simulink library "sm_trackV_lib_chain_contact_s46"  (R2026a)
settings: Solver=VariableStepAuto
undefined symbols (not defined in the file): Excv, L1, L10, L11, L12, L13, L14, L15, L16, L17, L18, L19, L2, L20, L21, L22, L23, L24, L25, L26, L27, L28, L29, L3, L30, L31, L32, L33, L34, L35, L36, L37, L38, L39, L4, L40, L41, L42, L43, L44, L45, L46, L5, L6, L7, L8, L9
libraries: sm_trackV_lib_chain_contact x276
Description:
  | Copyright 2024-2026 The MathWorks, Inc.
settings Model: Creator=smiller  LastModifiedBy=smiller

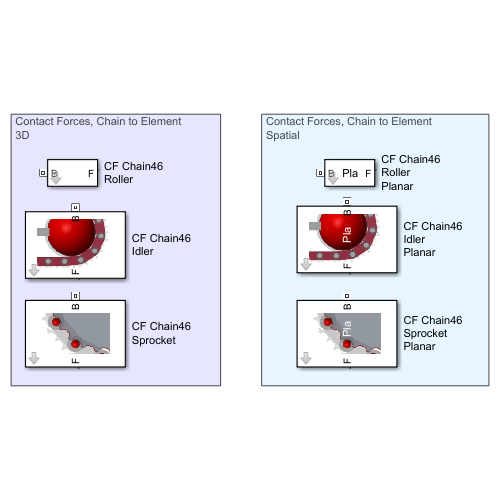
[thumbnail: Simulink's stored preview of the top-level diagram]
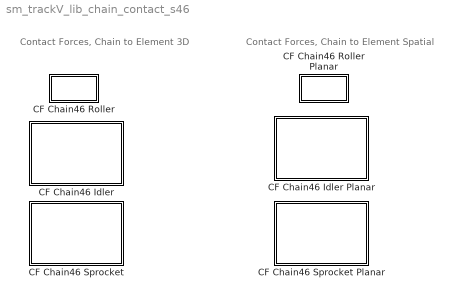
== system sm_trackV_lib_chain_contact_s46 ==
  note: Contact Forces, Chain to Element
      | 3D
  note: Contact Forces, Chain to Element
      | Spatial
  CF Chain46 Idler : Subsystem  mask(Contact Force, Full Chain to Idler){K_Idler=Excv.Contact.Idler.K, B_Idler=Excv.Contact.Idler.B, TW_Idler=Excv.Contact.Idler.TW}
      mask prompts: K_Idler "Normal Stiffness (N/m)"; B_Idler "Normal Damping (N/(m/s))"; TW_Idler "Normal Transition Width (m)"
      mask help: Models contact forces between entire chain and idler.
      mask Display: image('sm_excv_track_cf_chain_idler_IMAGE.png');
  CF Chain46 Idler Planar : Subsystem  mask(Contact Force, Full Chain to Idler){K_Idler=Excv.Contact.Idler.K, B_Idler=Excv.Contact.Idler.B, TW_Idler=Excv.Contact.Idler.TW}
      mask prompts: K_Idler "Normal Stiffness (N/m)"; B_Idler "Normal Damping (N/(m/s))"; TW_Idler "Normal Transition Width (m)"
      mask help: Models contact forces between entire chain and idler.
      mask Display:
      | image('sm_excv_track_cf_chain_idler_IMAGE.png');
      | color('white')
      | disp('   Pla');
  CF Chain46 Roller : Subsystem  mask(Contact Force, Full Chain to One Roller){K_Roller=Excv.Contact.Roller.K, B_Roller=Excv.Contact.Roller.B, TW_Roller=Excv.Contact.Roller.TW}
      mask prompts: K_Roller "Normal Stiffness (N/m)"; B_Roller "Normal Damping (N/(m/s))"; TW_Roller "Normal Transition Width (m)"
      mask help: Models contact forces between entire chain and one roller.
  CF Chain46 Roller Planar : Subsystem  mask(Contact Force, Full Chain to One Roller){K_Roller=Excv.Contact.Roller.K, B_Roller=Excv.Contact.Roller.B, TW_Roller=Excv.Contact.Roller.TW}
      mask prompts: K_Roller "Normal Stiffness (N/m)"; B_Roller "Normal Damping (N/(m/s))"; TW_Roller "Normal Transition Width (m)"
      mask help: Models contact forces between entire chain and one roller.
      mask Display: disp('Pla');
  CF Chain46 Sprocket : Subsystem  mask(Contact Force, Full Chain to Sprocket){K_Sprocket=Excv.Contact.Sprocket.K, B_Sprocket=Excv.Contact.Sprocket.B, TW_Sprocket=Excv.Contact.Sprocket.TW}
      mask prompts: K_Sprocket "Normal Stiffness (N/m)"; B_Sprocket "Normal Damping (N/(m/s))"; TW_Sprocket "Normal Transition Width (m)"
      mask help: Models contact forces between entire chain and sprocket.
      mask Display: image('sm_excv_track_cf_chain_teeth_IMAGE.png')
  CF Chain46 Sprocket Planar : Subsystem  mask(Contact Force, Full Chain to Sprocket){K_Sprocket=Excv.Contact.Sprocket.K, B_Sprocket=Excv.Contact.Sprocket.B, TW_Sprocket=Excv.Contact.Sprocket.TW}
      mask prompts: K_Sprocket "Normal Stiffness (N/m)"; B_Sprocket "Normal Damping (N/(m/s))"; TW_Sprocket "Normal Transition Width (m)"
      mask help: Models contact forces between entire chain and sprocket.
      mask Display:
      | image('sm_excv_track_cf_chain_teeth_IMAGE.png')
      | color('white')
      | disp('   Pla');

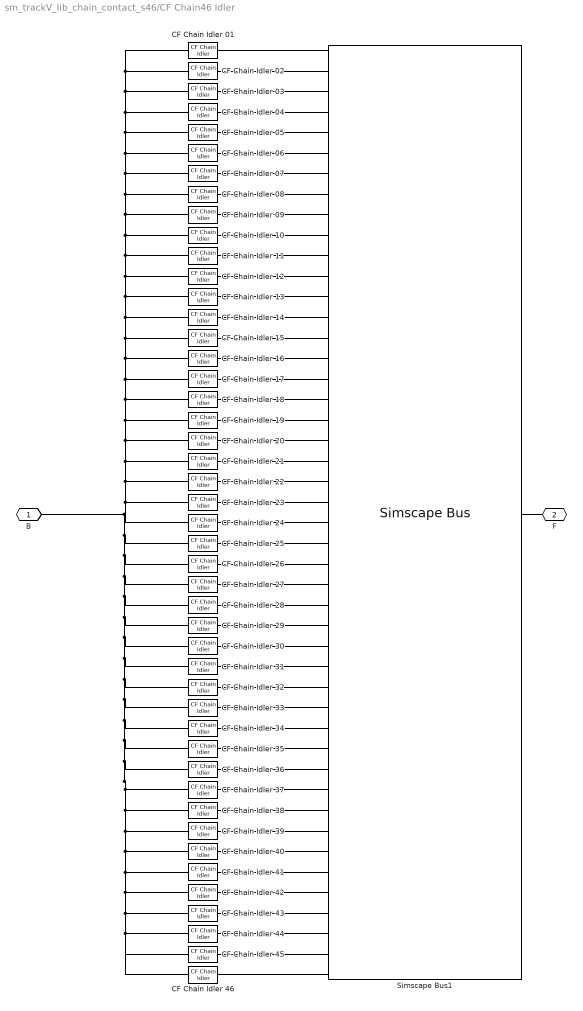
== system sm_trackV_lib_chain_contact_s46/CF Chain46 Idler ==
  CF Chain Idler 01 : sm_trackV_lib_chain_contact/CF Chain Idler  NormalStiffness=K_Idler  NormalDamping=B_Idler  NormalTransitionRegionWidth=TW_Idler
      settings: LibrarySourceBlock=sm_chain_drive_lib/CF_Idler
  CF Chain Idler 02 : sm_trackV_lib_chain_contact/CF Chain Idler  NormalStiffness=K_Idler  NormalDamping=B_Idler  NormalTransitionRegionWidth=TW_Idler
      settings: LibrarySourceBlock=sm_chain_drive_lib/CF_Idler
  CF Chain Idler 03 : sm_trackV_lib_chain_contact/CF Chain Idler  NormalStiffness=K_Idler  NormalDamping=B_Idler  NormalTransitionRegionWidth=TW_Idler
      settings: LibrarySourceBlock=sm_chain_drive_lib/CF_Idler
  CF Chain Idler 04 : sm_trackV_lib_chain_contact/CF Chain Idler  NormalStiffness=K_Idler  NormalDamping=B_Idler  NormalTransitionRegionWidth=TW_Idler
      settings: LibrarySourceBlock=sm_chain_drive_lib/CF_Idler
  CF Chain Idler 05 : sm_trackV_lib_chain_contact/CF Chain Idler  NormalStiffness=K_Idler  NormalDamping=B_Idler  NormalTransitionRegionWidth=TW_Idler
      settings: LibrarySourceBlock=sm_chain_drive_lib/CF_Idler
  CF Chain Idler 06 : sm_trackV_lib_chain_contact/CF Chain Idler  NormalStiffness=K_Idler  NormalDamping=B_Idler  NormalTransitionRegionWidth=TW_Idler
      settings: LibrarySourceBlock=sm_chain_drive_lib/CF_Idler
  CF Chain Idler 07 : sm_trackV_lib_chain_contact/CF Chain Idler  NormalStiffness=K_Idler  NormalDamping=B_Idler  NormalTransitionRegionWidth=TW_Idler
      settings: LibrarySourceBlock=sm_chain_drive_lib/CF_Idler
  CF Chain Idler 08 : sm_trackV_lib_chain_contact/CF Chain Idler  NormalStiffness=K_Idler  NormalDamping=B_Idler  NormalTransitionRegionWidth=TW_Idler
      settings: LibrarySourceBlock=sm_chain_drive_lib/CF_Idler
  CF Chain Idler 09 : sm_trackV_lib_chain_contact/CF Chain Idler  NormalStiffness=K_Idler  NormalDamping=B_Idler  NormalTransitionRegionWidth=TW_Idler
      settings: LibrarySourceBlock=sm_chain_drive_lib/CF_Idler
  CF Chain Idler {10..46} (37 alike) : sm_trackV_lib_chain_contact/CF Chain Idler  NormalStiffness=K_Idler  NormalDamping=B_Idler  NormalTransitionRegionWidth=TW_Idler
      settings: LibrarySourceBlock=sm_chain_drive_lib/CF_Idler
  Simscape Bus1 : SimscapeBus  HierarchyStrings=L1;L2;L3;L4;L5;L6;L7;L8;L9;L10;L11;L12;L13;L14;L15;L16;L17;L18;L19;L20;L21;L22;L23;L24;L25;L26;L27;L28;L29;L30;L31;L32;L33;L34;L35;L36;L37;L38;L39;L40;L41;L42;L43;L44;L45;L46  ConnectionType=Bus: CBO_Chain46
  B : PMIOPort  Side=Left
  F : PMIOPort  Port=2  Side=Right
  connections:
  Simscape Bus1/RConn1 -- F/RConn1
  Simscape Bus1/LConn28 -- CF Chain Idler 28/RConn1
  Simscape Bus1/LConn27 -- CF Chain Idler 27/RConn1
  Simscape Bus1/LConn26 -- CF Chain Idler 26/RConn1
  Simscape Bus1/LConn25 -- CF Chain Idler 25/RConn1
  Simscape Bus1/LConn24 -- CF Chain Idler 24/RConn1
  Simscape Bus1/LConn23 -- CF Chain Idler 23/RConn1
  Simscape Bus1/LConn22 -- CF Chain Idler 22/RConn1
  Simscape Bus1/LConn21 -- CF Chain Idler 21/RConn1
  Simscape Bus1/LConn20 -- CF Chain Idler 20/RConn1
  Simscape Bus1/LConn19 -- CF Chain Idler 19/RConn1
  Simscape Bus1/LConn18 -- CF Chain Idler 18/RConn1
  Simscape Bus1/LConn17 -- CF Chain Idler 17/RConn1
  Simscape Bus1/LConn16 -- CF Chain Idler 16/RConn1
  Simscape Bus1/LConn15 -- CF Chain Idler 15/RConn1
  Simscape Bus1/LConn14 -- CF Chain Idler 14/RConn1
  Simscape Bus1/LConn13 -- CF Chain Idler 13/RConn1
  Simscape Bus1/LConn12 -- CF Chain Idler 12/RConn1
  Simscape Bus1/LConn11 -- CF Chain Idler 11/RConn1
  Simscape Bus1/LConn10 -- CF Chain Idler 10/RConn1
  Simscape Bus1/LConn9 -- CF Chain Idler 09/RConn1
  Simscape Bus1/LConn8 -- CF Chain Idler 08/RConn1
  Simscape Bus1/LConn7 -- CF Chain Idler 07/RConn1
  Simscape Bus1/LConn6 -- CF Chain Idler 06/RConn1
  Simscape Bus1/LConn5 -- CF Chain Idler 05/RConn1
  Simscape Bus1/LConn4 -- CF Chain Idler 04/RConn1
  Simscape Bus1/LConn3 -- CF Chain Idler 03/RConn1
  Simscape Bus1/LConn2 -- CF Chain Idler 02/RConn1
  Simscape Bus1/LConn1 -- CF Chain Idler 01/RConn1
  CF Chain Idler 02/LConn1 -- CF Chain Idler 01/LConn1 -- CF Chain Idler 03/LConn1 -- CF Chain Idler 04/LConn1 -- CF Chain Idler 05/LConn1 -- CF Chain Idler 06/LConn1 -- CF Chain Idler 07/LConn1 -- CF Chain Idler 08/LConn1 -- CF Chain Idler 09/LConn1 -- CF Chain Idler 10/LConn1 -- CF Chain Idler 11/LConn1 -- CF Chain Idler 12/LConn1 -- CF Chain Idler 13/LConn1 -- CF Chain Idler 14/LConn1 -- CF Chain Idler 15/LConn1 -- CF Chain Idler 16/LConn1 -- CF Chain Idler 17/LConn1 -- CF Chain Idler 18/LConn1 -- CF Chain Idler 19/LConn1 -- CF Chain Idler 20/LConn1 -- CF Chain Idler 21/LConn1 -- CF Chain Idler 22/LConn1 -- CF Chain Idler 23/LConn1 -- B/RConn1 -- CF Chain Idler 24/LConn1 -- CF Chain Idler 25/LConn1 -- CF Chain Idler 26/LConn1 -- CF Chain Idler 27/LConn1 -- CF Chain Idler 28/LConn1 -- CF Chain Idler 29/LConn1 -- CF Chain Idler 30/LConn1 -- CF Chain Idler 31/LConn1 -- CF Chain Idler 32/LConn1 -- CF Chain Idler 33/LConn1 -- CF Chain Idler 34/LConn1 -- CF Chain Idler 35/LConn1 -- CF Chain Idler 36/LConn1 -- CF Chain Idler 37/LConn1 -- CF Chain Idler 38/LConn1 -- CF Chain Idler 39/LConn1 -- CF Chain Idler 40/LConn1 -- CF Chain Idler 41/LConn1 -- CF Chain Idler 42/LConn1 -- CF Chain Idler 43/LConn1 -- CF Chain Idler 44/LConn1 -- CF Chain Idler 46/LConn1 -- CF Chain Idler 45/LConn1
  Simscape Bus1/LConn46 -- CF Chain Idler 46/RConn1
  Simscape Bus1/LConn45 -- CF Chain Idler 45/RConn1
  Simscape Bus1/LConn44 -- CF Chain Idler 44/RConn1
  Simscape Bus1/LConn43 -- CF Chain Idler 43/RConn1
  Simscape Bus1/LConn42 -- CF Chain Idler 42/RConn1
  Simscape Bus1/LConn41 -- CF Chain Idler 41/RConn1
  Simscape Bus1/LConn40 -- CF Chain Idler 40/RConn1
  Simscape Bus1/LConn39 -- CF Chain Idler 39/RConn1
  Simscape Bus1/LConn38 -- CF Chain Idler 38/RConn1
  Simscape Bus1/LConn37 -- CF Chain Idler 37/RConn1
  Simscape Bus1/LConn36 -- CF Chain Idler 36/RConn1
  Simscape Bus1/LConn35 -- CF Chain Idler 35/RConn1
  Simscape Bus1/LConn34 -- CF Chain Idler 34/RConn1
  Simscape Bus1/LConn33 -- CF Chain Idler 33/RConn1
  Simscape Bus1/LConn32 -- CF Chain Idler 32/RConn1
  Simscape Bus1/LConn31 -- CF Chain Idler 31/RConn1
  Simscape Bus1/LConn30 -- CF Chain Idler 30/RConn1
  Simscape Bus1/LConn29 -- CF Chain Idler 29/RConn1

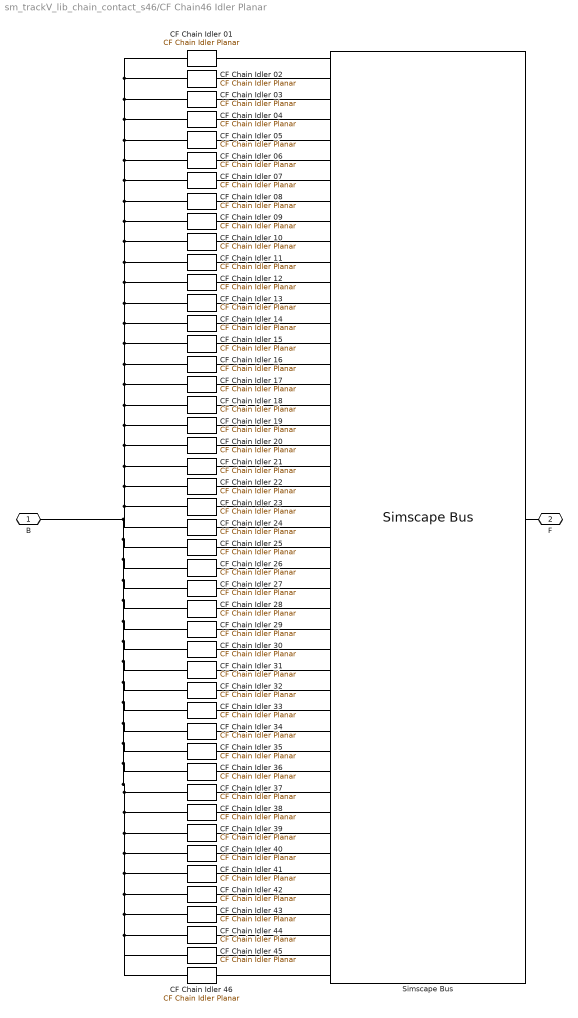
== system sm_trackV_lib_chain_contact_s46/CF Chain46 Idler Planar ==
  CF Chain Idler 01 : sm_trackV_lib_chain_contact/CF Chain Idler Planar  NormalStiffness=K_Idler  NormalDamping=B_Idler  NormalTransitionRegionWidth=TW_Idler
  CF Chain Idler 02 : sm_trackV_lib_chain_contact/CF Chain Idler Planar  NormalStiffness=K_Idler  NormalDamping=B_Idler  NormalTransitionRegionWidth=TW_Idler
  CF Chain Idler 03 : sm_trackV_lib_chain_contact/CF Chain Idler Planar  NormalStiffness=K_Idler  NormalDamping=B_Idler  NormalTransitionRegionWidth=TW_Idler
  CF Chain Idler 04 : sm_trackV_lib_chain_contact/CF Chain Idler Planar  NormalStiffness=K_Idler  NormalDamping=B_Idler  NormalTransitionRegionWidth=TW_Idler
  CF Chain Idler 05 : sm_trackV_lib_chain_contact/CF Chain Idler Planar  NormalStiffness=K_Idler  NormalDamping=B_Idler  NormalTransitionRegionWidth=TW_Idler
  CF Chain Idler 06 : sm_trackV_lib_chain_contact/CF Chain Idler Planar  NormalStiffness=K_Idler  NormalDamping=B_Idler  NormalTransitionRegionWidth=TW_Idler
  CF Chain Idler 07 : sm_trackV_lib_chain_contact/CF Chain Idler Planar  NormalStiffness=K_Idler  NormalDamping=B_Idler  NormalTransitionRegionWidth=TW_Idler
  CF Chain Idler 08 : sm_trackV_lib_chain_contact/CF Chain Idler Planar  NormalStiffness=K_Idler  NormalDamping=B_Idler  NormalTransitionRegionWidth=TW_Idler
  CF Chain Idler 09 : sm_trackV_lib_chain_contact/CF Chain Idler Planar  NormalStiffness=K_Idler  NormalDamping=B_Idler  NormalTransitionRegionWidth=TW_Idler
  CF Chain Idler {10..46} (37 alike) : sm_trackV_lib_chain_contact/CF Chain Idler Planar  NormalStiffness=K_Idler  NormalDamping=B_Idler  NormalTransitionRegionWidth=TW_Idler
  Simscape Bus : SimscapeBus  HierarchyStrings=L1;L2;L3;L4;L5;L6;L7;L8;L9;L10;L11;L12;L13;L14;L15;L16;L17;L18;L19;L20;L21;L22;L23;L24;L25;L26;L27;L28;L29;L30;L31;L32;L33;L34;L35;L36;L37;L38;L39;L40;L41;L42;L43;L44;L45;L46  ConnectionType=Bus: CBO_Chain46
  B : PMIOPort  Side=Left
  F : PMIOPort  Port=2  Side=Right
  connections:
  Simscape Bus/RConn1 -- F/RConn1
  CF Chain Idler 28/RConn1 -- Simscape Bus/LConn28
  CF Chain Idler 27/RConn1 -- Simscape Bus/LConn27
  CF Chain Idler 26/RConn1 -- Simscape Bus/LConn26
  CF Chain Idler 25/RConn1 -- Simscape Bus/LConn25
  CF Chain Idler 24/RConn1 -- Simscape Bus/LConn24
  CF Chain Idler 23/RConn1 -- Simscape Bus/LConn23
  CF Chain Idler 22/RConn1 -- Simscape Bus/LConn22
  CF Chain Idler 21/RConn1 -- Simscape Bus/LConn21
  CF Chain Idler 20/RConn1 -- Simscape Bus/LConn20
  CF Chain Idler 19/RConn1 -- Simscape Bus/LConn19
  CF Chain Idler 18/RConn1 -- Simscape Bus/LConn18
  CF Chain Idler 17/RConn1 -- Simscape Bus/LConn17
  CF Chain Idler 16/RConn1 -- Simscape Bus/LConn16
  CF Chain Idler 15/RConn1 -- Simscape Bus/LConn15
  CF Chain Idler 14/RConn1 -- Simscape Bus/LConn14
  CF Chain Idler 13/RConn1 -- Simscape Bus/LConn13
  CF Chain Idler 12/RConn1 -- Simscape Bus/LConn12
  CF Chain Idler 11/RConn1 -- Simscape Bus/LConn11
  CF Chain Idler 10/RConn1 -- Simscape Bus/LConn10
  CF Chain Idler 09/RConn1 -- Simscape Bus/LConn9
  CF Chain Idler 08/RConn1 -- Simscape Bus/LConn8
  CF Chain Idler 07/RConn1 -- Simscape Bus/LConn7
  CF Chain Idler 06/RConn1 -- Simscape Bus/LConn6
  CF Chain Idler 05/RConn1 -- Simscape Bus/LConn5
  CF Chain Idler 04/RConn1 -- Simscape Bus/LConn4
  CF Chain Idler 03/RConn1 -- Simscape Bus/LConn3
  CF Chain Idler 02/RConn1 -- Simscape Bus/LConn2
  CF Chain Idler 01/RConn1 -- Simscape Bus/LConn1
  CF Chain Idler 02/LConn1 -- CF Chain Idler 01/LConn1 -- CF Chain Idler 03/LConn1 -- CF Chain Idler 04/LConn1 -- CF Chain Idler 05/LConn1 -- CF Chain Idler 06/LConn1 -- CF Chain Idler 07/LConn1 -- CF Chain Idler 08/LConn1 -- CF Chain Idler 09/LConn1 -- CF Chain Idler 10/LConn1 -- CF Chain Idler 11/LConn1 -- CF Chain Idler 12/LConn1 -- CF Chain Idler 13/LConn1 -- CF Chain Idler 14/LConn1 -- CF Chain Idler 15/LConn1 -- CF Chain Idler 16/LConn1 -- CF Chain Idler 17/LConn1 -- CF Chain Idler 18/LConn1 -- CF Chain Idler 19/LConn1 -- CF Chain Idler 20/LConn1 -- CF Chain Idler 21/LConn1 -- CF Chain Idler 22/LConn1 -- CF Chain Idler 23/LConn1 -- B/RConn1 -- CF Chain Idler 24/LConn1 -- CF Chain Idler 25/LConn1 -- CF Chain Idler 26/LConn1 -- CF Chain Idler 27/LConn1 -- CF Chain Idler 28/LConn1 -- CF Chain Idler 29/LConn1 -- CF Chain Idler 30/LConn1 -- CF Chain Idler 31/LConn1 -- CF Chain Idler 32/LConn1 -- CF Chain Idler 33/LConn1 -- CF Chain Idler 34/LConn1 -- CF Chain Idler 35/LConn1 -- CF Chain Idler 36/LConn1 -- CF Chain Idler 37/LConn1 -- CF Chain Idler 38/LConn1 -- CF Chain Idler 39/LConn1 -- CF Chain Idler 40/LConn1 -- CF Chain Idler 41/LConn1 -- CF Chain Idler 42/LConn1 -- CF Chain Idler 43/LConn1 -- CF Chain Idler 44/LConn1 -- CF Chain Idler 46/LConn1 -- CF Chain Idler 45/LConn1
  CF Chain Idler 46/RConn1 -- Simscape Bus/LConn46
  CF Chain Idler 45/RConn1 -- Simscape Bus/LConn45
  CF Chain Idler 44/RConn1 -- Simscape Bus/LConn44
  CF Chain Idler 43/RConn1 -- Simscape Bus/LConn43
  CF Chain Idler 42/RConn1 -- Simscape Bus/LConn42
  CF Chain Idler 41/RConn1 -- Simscape Bus/LConn41
  CF Chain Idler 40/RConn1 -- Simscape Bus/LConn40
  CF Chain Idler 39/RConn1 -- Simscape Bus/LConn39
  CF Chain Idler 38/RConn1 -- Simscape Bus/LConn38
  CF Chain Idler 37/RConn1 -- Simscape Bus/LConn37
  CF Chain Idler 36/RConn1 -- Simscape Bus/LConn36
  CF Chain Idler 35/RConn1 -- Simscape Bus/LConn35
  CF Chain Idler 34/RConn1 -- Simscape Bus/LConn34
  CF Chain Idler 33/RConn1 -- Simscape Bus/LConn33
  CF Chain Idler 32/RConn1 -- Simscape Bus/LConn32
  CF Chain Idler 31/RConn1 -- Simscape Bus/LConn31
  CF Chain Idler 30/RConn1 -- Simscape Bus/LConn30
  CF Chain Idler 29/RConn1 -- Simscape Bus/LConn29

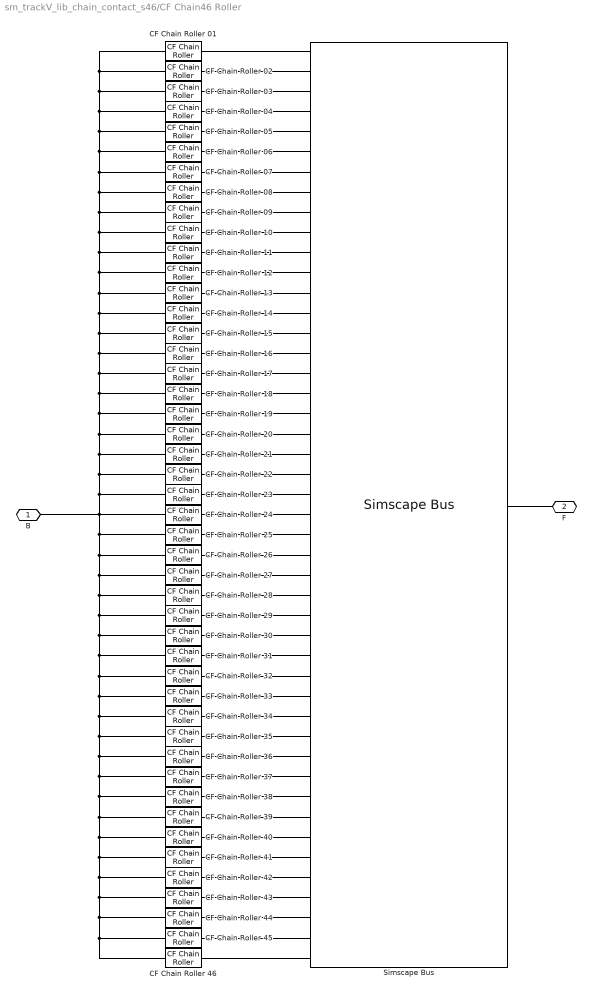
== system sm_trackV_lib_chain_contact_s46/CF Chain46 Roller ==
  CF Chain Roller 01 : sm_trackV_lib_chain_contact/CF Chain Roller  NormalStiffness=K_Roller  NormalDamping=B_Roller  NormalTransitionRegionWidth=TW_Roller
      settings: LibrarySourceBlock=sm_chain_drive_lib/CF_Pulley
  CF Chain Roller 02 : sm_trackV_lib_chain_contact/CF Chain Roller  NormalStiffness=K_Roller  NormalDamping=B_Roller  NormalTransitionRegionWidth=TW_Roller
      settings: LibrarySourceBlock=sm_chain_drive_lib/CF_Pulley
  CF Chain Roller 03 : sm_trackV_lib_chain_contact/CF Chain Roller  NormalStiffness=K_Roller  NormalDamping=B_Roller  NormalTransitionRegionWidth=TW_Roller
      settings: LibrarySourceBlock=sm_chain_drive_lib/CF_Pulley
  CF Chain Roller 04 : sm_trackV_lib_chain_contact/CF Chain Roller  NormalStiffness=K_Roller  NormalDamping=B_Roller  NormalTransitionRegionWidth=TW_Roller
      settings: LibrarySourceBlock=sm_chain_drive_lib/CF_Pulley
  CF Chain Roller 05 : sm_trackV_lib_chain_contact/CF Chain Roller  NormalStiffness=K_Roller  NormalDamping=B_Roller  NormalTransitionRegionWidth=TW_Roller
      settings: LibrarySourceBlock=sm_chain_drive_lib/CF_Pulley
  CF Chain Roller 06 : sm_trackV_lib_chain_contact/CF Chain Roller  NormalStiffness=K_Roller  NormalDamping=B_Roller  NormalTransitionRegionWidth=TW_Roller
      settings: LibrarySourceBlock=sm_chain_drive_lib/CF_Pulley
  CF Chain Roller 07 : sm_trackV_lib_chain_contact/CF Chain Roller  NormalStiffness=K_Roller  NormalDamping=B_Roller  NormalTransitionRegionWidth=TW_Roller
      settings: LibrarySourceBlock=sm_chain_drive_lib/CF_Pulley
  CF Chain Roller 08 : sm_trackV_lib_chain_contact/CF Chain Roller  NormalStiffness=K_Roller  NormalDamping=B_Roller  NormalTransitionRegionWidth=TW_Roller
      settings: LibrarySourceBlock=sm_chain_drive_lib/CF_Pulley
  CF Chain Roller 09 : sm_trackV_lib_chain_contact/CF Chain Roller  NormalStiffness=K_Roller  NormalDamping=B_Roller  NormalTransitionRegionWidth=TW_Roller
      settings: LibrarySourceBlock=sm_chain_drive_lib/CF_Pulley
  CF Chain Roller {10..46} (37 alike) : sm_trackV_lib_chain_contact/CF Chain Roller  NormalStiffness=K_Roller  NormalDamping=B_Roller  NormalTransitionRegionWidth=TW_Roller
      settings: LibrarySourceBlock=sm_chain_drive_lib/CF_Pulley
  Simscape Bus : SimscapeBus  HierarchyStrings=L1;L2;L3;L4;L5;L6;L7;L8;L9;L10;L11;L12;L13;L14;L15;L16;L17;L18;L19;L20;L21;L22;L23;L24;L25;L26;L27;L28;L29;L30;L31;L32;L33;L34;L35;L36;L37;L38;L39;L40;L41;L42;L43;L44;L45;L46  ConnectionType=Bus: CBO_Chain46
  B : PMIOPort  Side=Left
  F : PMIOPort  Port=2  Side=Right
  connections:
  CF Chain Roller 28/RConn1 -- Simscape Bus/LConn28
  CF Chain Roller 27/RConn1 -- Simscape Bus/LConn27
  CF Chain Roller 26/RConn1 -- Simscape Bus/LConn26
  CF Chain Roller 25/RConn1 -- Simscape Bus/LConn25
  CF Chain Roller 24/RConn1 -- Simscape Bus/LConn24
  CF Chain Roller 23/RConn1 -- Simscape Bus/LConn23
  CF Chain Roller 22/RConn1 -- Simscape Bus/LConn22
  CF Chain Roller 21/RConn1 -- Simscape Bus/LConn21
  CF Chain Roller 20/RConn1 -- Simscape Bus/LConn20
  CF Chain Roller 19/RConn1 -- Simscape Bus/LConn19
  CF Chain Roller 18/RConn1 -- Simscape Bus/LConn18
  CF Chain Roller 17/RConn1 -- Simscape Bus/LConn17
  CF Chain Roller 16/RConn1 -- Simscape Bus/LConn16
  CF Chain Roller 15/RConn1 -- Simscape Bus/LConn15
  CF Chain Roller 14/RConn1 -- Simscape Bus/LConn14
  CF Chain Roller 13/RConn1 -- Simscape Bus/LConn13
  CF Chain Roller 12/RConn1 -- Simscape Bus/LConn12
  CF Chain Roller 11/RConn1 -- Simscape Bus/LConn11
  CF Chain Roller 10/RConn1 -- Simscape Bus/LConn10
  CF Chain Roller 09/RConn1 -- Simscape Bus/LConn9
  CF Chain Roller 08/RConn1 -- Simscape Bus/LConn8
  CF Chain Roller 07/RConn1 -- Simscape Bus/LConn7
  CF Chain Roller 06/RConn1 -- Simscape Bus/LConn6
  CF Chain Roller 05/RConn1 -- Simscape Bus/LConn5
  CF Chain Roller 04/RConn1 -- Simscape Bus/LConn4
  CF Chain Roller 03/RConn1 -- Simscape Bus/LConn3
  CF Chain Roller 02/RConn1 -- Simscape Bus/LConn2
  Simscape Bus/LConn1 -- CF Chain Roller 01/RConn1
  Simscape Bus/RConn1 -- F/RConn1
  CF Chain Roller 29/RConn1 -- Simscape Bus/LConn29
  CF Chain Roller 30/RConn1 -- Simscape Bus/LConn30
  CF Chain Roller 31/RConn1 -- Simscape Bus/LConn31
  CF Chain Roller 32/RConn1 -- Simscape Bus/LConn32
  CF Chain Roller 33/RConn1 -- Simscape Bus/LConn33
  CF Chain Roller 34/RConn1 -- Simscape Bus/LConn34
  CF Chain Roller 35/RConn1 -- Simscape Bus/LConn35
  CF Chain Roller 36/RConn1 -- Simscape Bus/LConn36
  CF Chain Roller 37/RConn1 -- Simscape Bus/LConn37
  CF Chain Roller 38/RConn1 -- Simscape Bus/LConn38
  CF Chain Roller 39/RConn1 -- Simscape Bus/LConn39
  CF Chain Roller 40/RConn1 -- Simscape Bus/LConn40
  CF Chain Roller 41/RConn1 -- Simscape Bus/LConn41
  CF Chain Roller 42/RConn1 -- Simscape Bus/LConn42
  CF Chain Roller 43/RConn1 -- Simscape Bus/LConn43
  CF Chain Roller 44/RConn1 -- Simscape Bus/LConn44
  CF Chain Roller 45/RConn1 -- Simscape Bus/LConn45
  CF Chain Roller 46/RConn1 -- Simscape Bus/LConn46
  B/RConn1 -- CF Chain Roller 01/LConn1 -- CF Chain Roller 02/LConn1 -- CF Chain Roller 03/LConn1 -- CF Chain Roller 04/LConn1 -- CF Chain Roller 05/LConn1 -- CF Chain Roller 06/LConn1 -- CF Chain Roller 07/LConn1 -- CF Chain Roller 08/LConn1 -- CF Chain Roller 09/LConn1 -- CF Chain Roller 10/LConn1 -- CF Chain Roller 11/LConn1 -- CF Chain Roller 12/LConn1 -- CF Chain Roller 13/LConn1 -- CF Chain Roller 14/LConn1 -- CF Chain Roller 15/LConn1 -- CF Chain Roller 16/LConn1 -- CF Chain Roller 17/LConn1 -- CF Chain Roller 18/LConn1 -- CF Chain Roller 19/LConn1 -- CF Chain Roller 20/LConn1 -- CF Chain Roller 21/LConn1 -- CF Chain Roller 22/LConn1 -- CF Chain Roller 23/LConn1 -- CF Chain Roller 24/LConn1 -- CF Chain Roller 25/LConn1 -- CF Chain Roller 26/LConn1 -- CF Chain Roller 27/LConn1 -- CF Chain Roller 28/LConn1 -- CF Chain Roller 29/LConn1 -- CF Chain Roller 30/LConn1 -- CF Chain Roller 31/LConn1 -- CF Chain Roller 32/LConn1 -- CF Chain Roller 33/LConn1 -- CF Chain Roller 34/LConn1 -- CF Chain Roller 35/LConn1 -- CF Chain Roller 36/LConn1 -- CF Chain Roller 37/LConn1 -- CF Chain Roller 38/LConn1 -- CF Chain Roller 39/LConn1 -- CF Chain Roller 40/LConn1 -- CF Chain Roller 41/LConn1 -- CF Chain Roller 42/LConn1 -- CF Chain Roller 43/LConn1 -- CF Chain Roller 44/LConn1 -- CF Chain Roller 46/LConn1 -- CF Chain Roller 45/LConn1

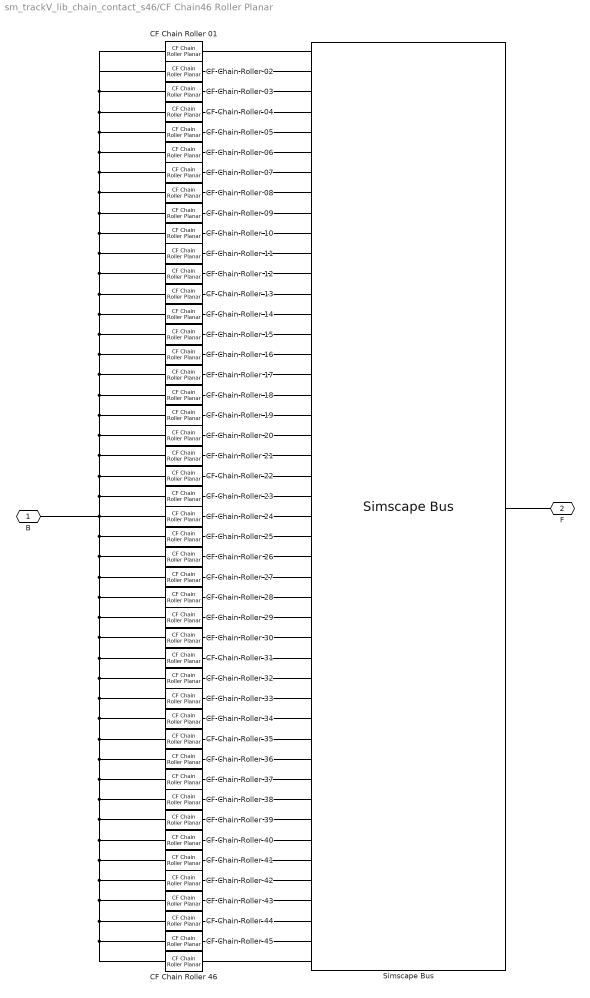
== system sm_trackV_lib_chain_contact_s46/CF Chain46 Roller Planar ==
  CF Chain Roller 01 : sm_trackV_lib_chain_contact/CF Chain Roller Planar  NormalStiffness=K_Roller  NormalDamping=B_Roller  NormalTransitionRegionWidth=TW_Roller
  CF Chain Roller 02 : sm_trackV_lib_chain_contact/CF Chain Roller Planar  NormalStiffness=K_Roller  NormalDamping=B_Roller  NormalTransitionRegionWidth=TW_Roller
  CF Chain Roller 03 : sm_trackV_lib_chain_contact/CF Chain Roller Planar  NormalStiffness=K_Roller  NormalDamping=B_Roller  NormalTransitionRegionWidth=TW_Roller
  CF Chain Roller 04 : sm_trackV_lib_chain_contact/CF Chain Roller Planar  NormalStiffness=K_Roller  NormalDamping=B_Roller  NormalTransitionRegionWidth=TW_Roller
  CF Chain Roller 05 : sm_trackV_lib_chain_contact/CF Chain Roller Planar  NormalStiffness=K_Roller  NormalDamping=B_Roller  NormalTransitionRegionWidth=TW_Roller
  CF Chain Roller 06 : sm_trackV_lib_chain_contact/CF Chain Roller Planar  NormalStiffness=K_Roller  NormalDamping=B_Roller  NormalTransitionRegionWidth=TW_Roller
  CF Chain Roller 07 : sm_trackV_lib_chain_contact/CF Chain Roller Planar  NormalStiffness=K_Roller  NormalDamping=B_Roller  NormalTransitionRegionWidth=TW_Roller
  CF Chain Roller 08 : sm_trackV_lib_chain_contact/CF Chain Roller Planar  NormalStiffness=K_Roller  NormalDamping=B_Roller  NormalTransitionRegionWidth=TW_Roller
  CF Chain Roller 09 : sm_trackV_lib_chain_contact/CF Chain Roller Planar  NormalStiffness=K_Roller  NormalDamping=B_Roller  NormalTransitionRegionWidth=TW_Roller
  CF Chain Roller {10..46} (37 alike) : sm_trackV_lib_chain_contact/CF Chain Roller Planar  NormalStiffness=K_Roller  NormalDamping=B_Roller  NormalTransitionRegionWidth=TW_Roller
  Simscape Bus : SimscapeBus  HierarchyStrings=L1;L2;L3;L4;L5;L6;L7;L8;L9;L10;L11;L12;L13;L14;L15;L16;L17;L18;L19;L20;L21;L22;L23;L24;L25;L26;L27;L28;L29;L30;L31;L32;L33;L34;L35;L36;L37;L38;L39;L40;L41;L42;L43;L44;L45;L46  ConnectionType=Bus: CBO_Chain46
  B : PMIOPort  Side=Left
  F : PMIOPort  Port=2  Side=Right
  connections:
  CF Chain Roller 45/LConn1 -- CF Chain Roller 46/LConn1 -- CF Chain Roller 44/LConn1 -- CF Chain Roller 43/LConn1 -- CF Chain Roller 42/LConn1 -- CF Chain Roller 41/LConn1 -- CF Chain Roller 40/LConn1 -- CF Chain Roller 39/LConn1 -- CF Chain Roller 38/LConn1 -- CF Chain Roller 37/LConn1 -- CF Chain Roller 36/LConn1 -- CF Chain Roller 35/LConn1 -- CF Chain Roller 34/LConn1 -- CF Chain Roller 33/LConn1 -- CF Chain Roller 32/LConn1 -- CF Chain Roller 31/LConn1 -- CF Chain Roller 30/LConn1 -- CF Chain Roller 29/LConn1 -- CF Chain Roller 28/LConn1 -- CF Chain Roller 27/LConn1 -- CF Chain Roller 26/LConn1 -- CF Chain Roller 25/LConn1 -- CF Chain Roller 24/LConn1 -- CF Chain Roller 23/LConn1 -- CF Chain Roller 22/LConn1 -- CF Chain Roller 21/LConn1 -- CF Chain Roller 20/LConn1 -- CF Chain Roller 19/LConn1 -- CF Chain Roller 18/LConn1 -- CF Chain Roller 17/LConn1 -- CF Chain Roller 16/LConn1 -- CF Chain Roller 15/LConn1 -- CF Chain Roller 14/LConn1 -- CF Chain Roller 13/LConn1 -- CF Chain Roller 12/LConn1 -- CF Chain Roller 11/LConn1 -- CF Chain Roller 10/LConn1 -- CF Chain Roller 09/LConn1 -- CF Chain Roller 08/LConn1 -- CF Chain Roller 07/LConn1 -- CF Chain Roller 06/LConn1 -- CF Chain Roller 05/LConn1 -- CF Chain Roller 04/LConn1 -- CF Chain Roller 03/LConn1 -- CF Chain Roller 02/LConn1 -- CF Chain Roller 01/LConn1 -- B/RConn1
  CF Chain Roller 46/RConn1 -- Simscape Bus/LConn46
  CF Chain Roller 45/RConn1 -- Simscape Bus/LConn45
  CF Chain Roller 44/RConn1 -- Simscape Bus/LConn44
  CF Chain Roller 43/RConn1 -- Simscape Bus/LConn43
  CF Chain Roller 42/RConn1 -- Simscape Bus/LConn42
  CF Chain Roller 41/RConn1 -- Simscape Bus/LConn41
  CF Chain Roller 40/RConn1 -- Simscape Bus/LConn40
  CF Chain Roller 39/RConn1 -- Simscape Bus/LConn39
  CF Chain Roller 38/RConn1 -- Simscape Bus/LConn38
  CF Chain Roller 37/RConn1 -- Simscape Bus/LConn37
  CF Chain Roller 36/RConn1 -- Simscape Bus/LConn36
  CF Chain Roller 35/RConn1 -- Simscape Bus/LConn35
  CF Chain Roller 34/RConn1 -- Simscape Bus/LConn34
  CF Chain Roller 33/RConn1 -- Simscape Bus/LConn33
  CF Chain Roller 32/RConn1 -- Simscape Bus/LConn32
  CF Chain Roller 31/RConn1 -- Simscape Bus/LConn31
  CF Chain Roller 30/RConn1 -- Simscape Bus/LConn30
  CF Chain Roller 29/RConn1 -- Simscape Bus/LConn29
  Simscape Bus/RConn1 -- F/RConn1
  Simscape Bus/LConn1 -- CF Chain Roller 01/RConn1
  CF Chain Roller 02/RConn1 -- Simscape Bus/LConn2
  CF Chain Roller 03/RConn1 -- Simscape Bus/LConn3
  CF Chain Roller 04/RConn1 -- Simscape Bus/LConn4
  CF Chain Roller 05/RConn1 -- Simscape Bus/LConn5
  CF Chain Roller 06/RConn1 -- Simscape Bus/LConn6
  CF Chain Roller 07/RConn1 -- Simscape Bus/LConn7
  CF Chain Roller 08/RConn1 -- Simscape Bus/LConn8
  CF Chain Roller 09/RConn1 -- Simscape Bus/LConn9
  CF Chain Roller 10/RConn1 -- Simscape Bus/LConn10
  CF Chain Roller 11/RConn1 -- Simscape Bus/LConn11
  CF Chain Roller 12/RConn1 -- Simscape Bus/LConn12
  CF Chain Roller 13/RConn1 -- Simscape Bus/LConn13
  CF Chain Roller 14/RConn1 -- Simscape Bus/LConn14
  CF Chain Roller 15/RConn1 -- Simscape Bus/LConn15
  CF Chain Roller 16/RConn1 -- Simscape Bus/LConn16
  CF Chain Roller 17/RConn1 -- Simscape Bus/LConn17
  CF Chain Roller 18/RConn1 -- Simscape Bus/LConn18
  CF Chain Roller 19/RConn1 -- Simscape Bus/LConn19
  CF Chain Roller 20/RConn1 -- Simscape Bus/LConn20
  CF Chain Roller 21/RConn1 -- Simscape Bus/LConn21
  CF Chain Roller 22/RConn1 -- Simscape Bus/LConn22
  CF Chain Roller 23/RConn1 -- Simscape Bus/LConn23
  CF Chain Roller 24/RConn1 -- Simscape Bus/LConn24
  CF Chain Roller 25/RConn1 -- Simscape Bus/LConn25
  CF Chain Roller 26/RConn1 -- Simscape Bus/LConn26
  CF Chain Roller 27/RConn1 -- Simscape Bus/LConn27
  CF Chain Roller 28/RConn1 -- Simscape Bus/LConn28

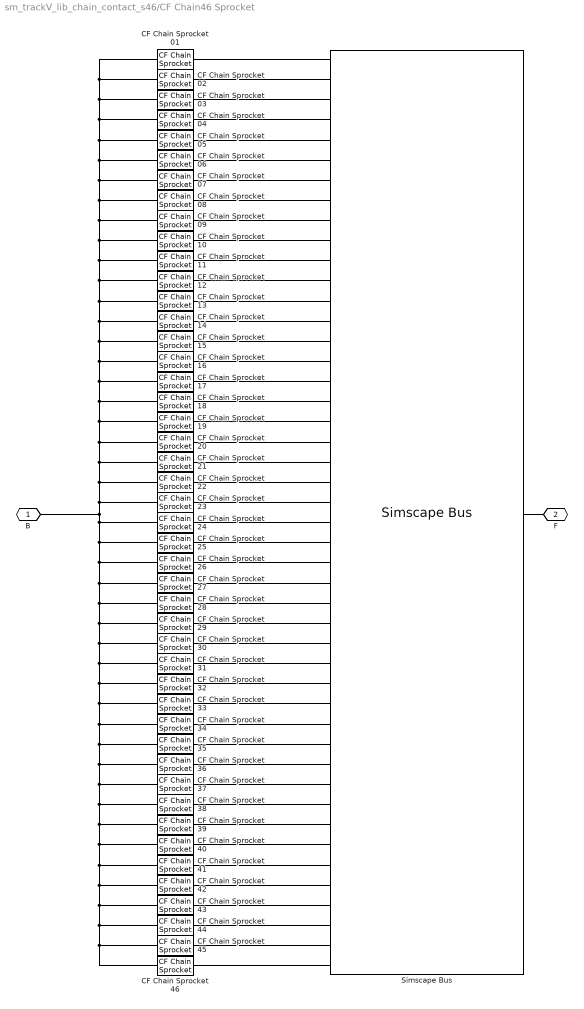
== system sm_trackV_lib_chain_contact_s46/CF Chain46 Sprocket ==
  CF Chain Sprocket 01 : sm_trackV_lib_chain_contact/CF Chain Sprocket  NormalStiffness=K_Sprocket  NormalDamping=B_Sprocket  NormalTransitionRegionWidth=TW_Sprocket
  CF Chain Sprocket 02 : sm_trackV_lib_chain_contact/CF Chain Sprocket  NormalStiffness=K_Sprocket  NormalDamping=B_Sprocket  NormalTransitionRegionWidth=TW_Sprocket
  CF Chain Sprocket 03 : sm_trackV_lib_chain_contact/CF Chain Sprocket  NormalStiffness=K_Sprocket  NormalDamping=B_Sprocket  NormalTransitionRegionWidth=TW_Sprocket
  CF Chain Sprocket 04 : sm_trackV_lib_chain_contact/CF Chain Sprocket  NormalStiffness=K_Sprocket  NormalDamping=B_Sprocket  NormalTransitionRegionWidth=TW_Sprocket
  CF Chain Sprocket 05 : sm_trackV_lib_chain_contact/CF Chain Sprocket  NormalStiffness=K_Sprocket  NormalDamping=B_Sprocket  NormalTransitionRegionWidth=TW_Sprocket
  CF Chain Sprocket 06 : sm_trackV_lib_chain_contact/CF Chain Sprocket  NormalStiffness=K_Sprocket  NormalDamping=B_Sprocket  NormalTransitionRegionWidth=TW_Sprocket
  CF Chain Sprocket 07 : sm_trackV_lib_chain_contact/CF Chain Sprocket  NormalStiffness=K_Sprocket  NormalDamping=B_Sprocket  NormalTransitionRegionWidth=TW_Sprocket
  CF Chain Sprocket 08 : sm_trackV_lib_chain_contact/CF Chain Sprocket  NormalStiffness=K_Sprocket  NormalDamping=B_Sprocket  NormalTransitionRegionWidth=TW_Sprocket
  CF Chain Sprocket 09 : sm_trackV_lib_chain_contact/CF Chain Sprocket  NormalStiffness=K_Sprocket  NormalDamping=B_Sprocket  NormalTransitionRegionWidth=TW_Sprocket
  CF Chain Sprocket {10..46} (37 alike) : sm_trackV_lib_chain_contact/CF Chain Sprocket  NormalStiffness=K_Sprocket  NormalDamping=B_Sprocket  NormalTransitionRegionWidth=TW_Sprocket
  Simscape Bus : SimscapeBus  HierarchyStrings=L1;L2;L3;L4;L5;L6;L7;L8;L9;L10;L11;L12;L13;L14;L15;L16;L17;L18;L19;L20;L21;L22;L23;L24;L25;L26;L27;L28;L29;L30;L31;L32;L33;L34;L35;L36;L37;L38;L39;L40;L41;L42;L43;L44;L45;L46  ConnectionType=Bus: CBO_Chain46
  B : PMIOPort  Side=Left
  F : PMIOPort  Port=2  Side=Right
  connections:
  CF Chain Sprocket 29/RConn1 -- Simscape Bus/LConn29
  CF Chain Sprocket 30/RConn1 -- Simscape Bus/LConn30
  CF Chain Sprocket 31/RConn1 -- Simscape Bus/LConn31
  CF Chain Sprocket 32/RConn1 -- Simscape Bus/LConn32
  CF Chain Sprocket 33/RConn1 -- Simscape Bus/LConn33
  CF Chain Sprocket 34/RConn1 -- Simscape Bus/LConn34
  CF Chain Sprocket 35/RConn1 -- Simscape Bus/LConn35
  CF Chain Sprocket 36/RConn1 -- Simscape Bus/LConn36
  CF Chain Sprocket 37/RConn1 -- Simscape Bus/LConn37
  CF Chain Sprocket 38/RConn1 -- Simscape Bus/LConn38
  CF Chain Sprocket 39/RConn1 -- Simscape Bus/LConn39
  CF Chain Sprocket 40/RConn1 -- Simscape Bus/LConn40
  CF Chain Sprocket 41/RConn1 -- Simscape Bus/LConn41
  CF Chain Sprocket 42/RConn1 -- Simscape Bus/LConn42
  CF Chain Sprocket 43/RConn1 -- Simscape Bus/LConn43
  CF Chain Sprocket 44/RConn1 -- Simscape Bus/LConn44
  CF Chain Sprocket 45/RConn1 -- Simscape Bus/LConn45
  CF Chain Sprocket 46/RConn1 -- Simscape Bus/LConn46
  CF Chain Sprocket 46/LConn1 -- CF Chain Sprocket 45/LConn1 -- CF Chain Sprocket 44/LConn1 -- CF Chain Sprocket 43/LConn1 -- CF Chain Sprocket 42/LConn1 -- CF Chain Sprocket 41/LConn1 -- CF Chain Sprocket 40/LConn1 -- CF Chain Sprocket 39/LConn1 -- CF Chain Sprocket 38/LConn1 -- CF Chain Sprocket 37/LConn1 -- B/RConn1 -- CF Chain Sprocket 01/LConn1 -- CF Chain Sprocket 02/LConn1 -- CF Chain Sprocket 03/LConn1 -- CF Chain Sprocket 04/LConn1 -- CF Chain Sprocket 05/LConn1 -- CF Chain Sprocket 06/LConn1 -- CF Chain Sprocket 07/LConn1 -- CF Chain Sprocket 08/LConn1 -- CF Chain Sprocket 09/LConn1 -- CF Chain Sprocket 10/LConn1 -- CF Chain Sprocket 11/LConn1 -- CF Chain Sprocket 12/LConn1 -- CF Chain Sprocket 13/LConn1 -- CF Chain Sprocket 14/LConn1 -- CF Chain Sprocket 15/LConn1 -- CF Chain Sprocket 16/LConn1 -- CF Chain Sprocket 17/LConn1 -- CF Chain Sprocket 18/LConn1 -- CF Chain Sprocket 19/LConn1 -- CF Chain Sprocket 20/LConn1 -- CF Chain Sprocket 21/LConn1 -- CF Chain Sprocket 22/LConn1 -- CF Chain Sprocket 23/LConn1 -- CF Chain Sprocket 24/LConn1 -- CF Chain Sprocket 25/LConn1 -- CF Chain Sprocket 26/LConn1 -- CF Chain Sprocket 27/LConn1 -- CF Chain Sprocket 28/LConn1 -- CF Chain Sprocket 29/LConn1 -- CF Chain Sprocket 30/LConn1 -- CF Chain Sprocket 31/LConn1 -- CF Chain Sprocket 32/LConn1 -- CF Chain Sprocket 33/LConn1 -- CF Chain Sprocket 34/LConn1 -- CF Chain Sprocket 35/LConn1 -- CF Chain Sprocket 36/LConn1
  CF Chain Sprocket 01/RConn1 -- Simscape Bus/LConn1
  CF Chain Sprocket 02/RConn1 -- Simscape Bus/LConn2
  CF Chain Sprocket 03/RConn1 -- Simscape Bus/LConn3
  CF Chain Sprocket 04/RConn1 -- Simscape Bus/LConn4
  CF Chain Sprocket 05/RConn1 -- Simscape Bus/LConn5
  CF Chain Sprocket 06/RConn1 -- Simscape Bus/LConn6
  CF Chain Sprocket 07/RConn1 -- Simscape Bus/LConn7
  CF Chain Sprocket 08/RConn1 -- Simscape Bus/LConn8
  CF Chain Sprocket 09/RConn1 -- Simscape Bus/LConn9
  CF Chain Sprocket 10/RConn1 -- Simscape Bus/LConn10
  CF Chain Sprocket 11/RConn1 -- Simscape Bus/LConn11
  CF Chain Sprocket 12/RConn1 -- Simscape Bus/LConn12
  CF Chain Sprocket 13/RConn1 -- Simscape Bus/LConn13
  CF Chain Sprocket 14/RConn1 -- Simscape Bus/LConn14
  CF Chain Sprocket 15/RConn1 -- Simscape Bus/LConn15
  CF Chain Sprocket 16/RConn1 -- Simscape Bus/LConn16
  CF Chain Sprocket 17/RConn1 -- Simscape Bus/LConn17
  CF Chain Sprocket 18/RConn1 -- Simscape Bus/LConn18
  CF Chain Sprocket 19/RConn1 -- Simscape Bus/LConn19
  CF Chain Sprocket 20/RConn1 -- Simscape Bus/LConn20
  CF Chain Sprocket 21/RConn1 -- Simscape Bus/LConn21
  CF Chain Sprocket 22/RConn1 -- Simscape Bus/LConn22
  CF Chain Sprocket 23/RConn1 -- Simscape Bus/LConn23
  CF Chain Sprocket 24/RConn1 -- Simscape Bus/LConn24
  CF Chain Sprocket 25/RConn1 -- Simscape Bus/LConn25
  CF Chain Sprocket 26/RConn1 -- Simscape Bus/LConn26
  CF Chain Sprocket 27/RConn1 -- Simscape Bus/LConn27
  CF Chain Sprocket 28/RConn1 -- Simscape Bus/LConn28
  Simscape Bus/RConn1 -- F/RConn1

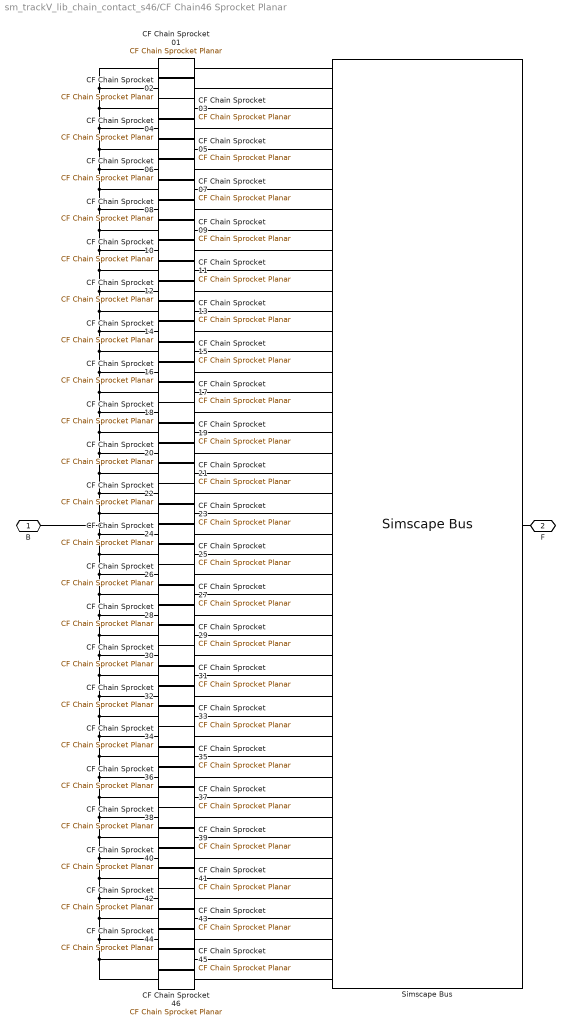
== system sm_trackV_lib_chain_contact_s46/CF Chain46 Sprocket Planar ==
  CF Chain Sprocket 01 : sm_trackV_lib_chain_contact/CF Chain Sprocket Planar  NormalStiffness=K_Sprocket  NormalDamping=B_Sprocket  NormalTransitionRegionWidth=TW_Sprocket
  CF Chain Sprocket 02 : sm_trackV_lib_chain_contact/CF Chain Sprocket Planar  NormalStiffness=K_Sprocket  NormalDamping=B_Sprocket  NormalTransitionRegionWidth=TW_Sprocket
  CF Chain Sprocket 03 : sm_trackV_lib_chain_contact/CF Chain Sprocket Planar  NormalStiffness=K_Sprocket  NormalDamping=B_Sprocket  NormalTransitionRegionWidth=TW_Sprocket
  CF Chain Sprocket 04 : sm_trackV_lib_chain_contact/CF Chain Sprocket Planar  NormalStiffness=K_Sprocket  NormalDamping=B_Sprocket  NormalTransitionRegionWidth=TW_Sprocket
  CF Chain Sprocket 05 : sm_trackV_lib_chain_contact/CF Chain Sprocket Planar  NormalStiffness=K_Sprocket  NormalDamping=B_Sprocket  NormalTransitionRegionWidth=TW_Sprocket
  CF Chain Sprocket 06 : sm_trackV_lib_chain_contact/CF Chain Sprocket Planar  NormalStiffness=K_Sprocket  NormalDamping=B_Sprocket  NormalTransitionRegionWidth=TW_Sprocket
  CF Chain Sprocket 07 : sm_trackV_lib_chain_contact/CF Chain Sprocket Planar  NormalStiffness=K_Sprocket  NormalDamping=B_Sprocket  NormalTransitionRegionWidth=TW_Sprocket
  CF Chain Sprocket 08 : sm_trackV_lib_chain_contact/CF Chain Sprocket Planar  NormalStiffness=K_Sprocket  NormalDamping=B_Sprocket  NormalTransitionRegionWidth=TW_Sprocket
  CF Chain Sprocket 09 : sm_trackV_lib_chain_contact/CF Chain Sprocket Planar  NormalStiffness=K_Sprocket  NormalDamping=B_Sprocket  NormalTransitionRegionWidth=TW_Sprocket
  CF Chain Sprocket {10..46} (37 alike) : sm_trackV_lib_chain_contact/CF Chain Sprocket Planar  NormalStiffness=K_Sprocket  NormalDamping=B_Sprocket  NormalTransitionRegionWidth=TW_Sprocket
  Simscape Bus : SimscapeBus  HierarchyStrings=L1;L2;L3;L4;L5;L6;L7;L8;L9;L10;L11;L12;L13;L14;L15;L16;L17;L18;L19;L20;L21;L22;L23;L24;L25;L26;L27;L28;L29;L30;L31;L32;L33;L34;L35;L36;L37;L38;L39;L40;L41;L42;L43;L44;L45;L46  ConnectionType=Bus: CBO_Chain46
  B : PMIOPort  Side=Left
  F : PMIOPort  Port=2  Side=Right
  connections:
  CF Chain Sprocket 29/RConn1 -- Simscape Bus/LConn29
  CF Chain Sprocket 30/RConn1 -- Simscape Bus/LConn30
  CF Chain Sprocket 31/RConn1 -- Simscape Bus/LConn31
  CF Chain Sprocket 32/RConn1 -- Simscape Bus/LConn32
  CF Chain Sprocket 33/RConn1 -- Simscape Bus/LConn33
  CF Chain Sprocket 34/RConn1 -- Simscape Bus/LConn34
  CF Chain Sprocket 35/RConn1 -- Simscape Bus/LConn35
  CF Chain Sprocket 36/RConn1 -- Simscape Bus/LConn36
  CF Chain Sprocket 37/RConn1 -- Simscape Bus/LConn37
  CF Chain Sprocket 38/RConn1 -- Simscape Bus/LConn38
  CF Chain Sprocket 39/RConn1 -- Simscape Bus/LConn39
  CF Chain Sprocket 40/RConn1 -- Simscape Bus/LConn40
  CF Chain Sprocket 41/RConn1 -- Simscape Bus/LConn41
  CF Chain Sprocket 42/RConn1 -- Simscape Bus/LConn42
  CF Chain Sprocket 43/RConn1 -- Simscape Bus/LConn43
  CF Chain Sprocket 44/RConn1 -- Simscape Bus/LConn44
  CF Chain Sprocket 45/RConn1 -- Simscape Bus/LConn45
  CF Chain Sprocket 46/RConn1 -- Simscape Bus/LConn46
  CF Chain Sprocket 46/LConn1 -- CF Chain Sprocket 45/LConn1 -- CF Chain Sprocket 44/LConn1 -- CF Chain Sprocket 43/LConn1 -- CF Chain Sprocket 42/LConn1 -- CF Chain Sprocket 41/LConn1 -- CF Chain Sprocket 40/LConn1 -- CF Chain Sprocket 39/LConn1 -- CF Chain Sprocket 38/LConn1 -- CF Chain Sprocket 37/LConn1 -- B/RConn1 -- CF Chain Sprocket 01/LConn1 -- CF Chain Sprocket 02/LConn1 -- CF Chain Sprocket 03/LConn1 -- CF Chain Sprocket 04/LConn1 -- CF Chain Sprocket 05/LConn1 -- CF Chain Sprocket 06/LConn1 -- CF Chain Sprocket 07/LConn1 -- CF Chain Sprocket 08/LConn1 -- CF Chain Sprocket 09/LConn1 -- CF Chain Sprocket 10/LConn1 -- CF Chain Sprocket 11/LConn1 -- CF Chain Sprocket 12/LConn1 -- CF Chain Sprocket 13/LConn1 -- CF Chain Sprocket 14/LConn1 -- CF Chain Sprocket 15/LConn1 -- CF Chain Sprocket 16/LConn1 -- CF Chain Sprocket 17/LConn1 -- CF Chain Sprocket 18/LConn1 -- CF Chain Sprocket 19/LConn1 -- CF Chain Sprocket 20/LConn1 -- CF Chain Sprocket 21/LConn1 -- CF Chain Sprocket 22/LConn1 -- CF Chain Sprocket 23/LConn1 -- CF Chain Sprocket 24/LConn1 -- CF Chain Sprocket 25/LConn1 -- CF Chain Sprocket 26/LConn1 -- CF Chain Sprocket 27/LConn1 -- CF Chain Sprocket 28/LConn1 -- CF Chain Sprocket 29/LConn1 -- CF Chain Sprocket 30/LConn1 -- CF Chain Sprocket 31/LConn1 -- CF Chain Sprocket 32/LConn1 -- CF Chain Sprocket 33/LConn1 -- CF Chain Sprocket 34/LConn1 -- CF Chain Sprocket 35/LConn1 -- CF Chain Sprocket 36/LConn1
  CF Chain Sprocket 01/RConn1 -- Simscape Bus/LConn1
  CF Chain Sprocket 02/RConn1 -- Simscape Bus/LConn2
  CF Chain Sprocket 03/RConn1 -- Simscape Bus/LConn3
  CF Chain Sprocket 04/RConn1 -- Simscape Bus/LConn4
  CF Chain Sprocket 05/RConn1 -- Simscape Bus/LConn5
  CF Chain Sprocket 06/RConn1 -- Simscape Bus/LConn6
  CF Chain Sprocket 07/RConn1 -- Simscape Bus/LConn7
  CF Chain Sprocket 08/RConn1 -- Simscape Bus/LConn8
  CF Chain Sprocket 09/RConn1 -- Simscape Bus/LConn9
  CF Chain Sprocket 10/RConn1 -- Simscape Bus/LConn10
  CF Chain Sprocket 11/RConn1 -- Simscape Bus/LConn11
  CF Chain Sprocket 12/RConn1 -- Simscape Bus/LConn12
  CF Chain Sprocket 13/RConn1 -- Simscape Bus/LConn13
  CF Chain Sprocket 14/RConn1 -- Simscape Bus/LConn14
  CF Chain Sprocket 15/RConn1 -- Simscape Bus/LConn15
  CF Chain Sprocket 16/RConn1 -- Simscape Bus/LConn16
  CF Chain Sprocket 17/RConn1 -- Simscape Bus/LConn17
  CF Chain Sprocket 18/RConn1 -- Simscape Bus/LConn18
  CF Chain Sprocket 19/RConn1 -- Simscape Bus/LConn19
  CF Chain Sprocket 20/RConn1 -- Simscape Bus/LConn20
  CF Chain Sprocket 21/RConn1 -- Simscape Bus/LConn21
  CF Chain Sprocket 22/RConn1 -- Simscape Bus/LConn22
  CF Chain Sprocket 23/RConn1 -- Simscape Bus/LConn23
  CF Chain Sprocket 24/RConn1 -- Simscape Bus/LConn24
  CF Chain Sprocket 25/RConn1 -- Simscape Bus/LConn25
  CF Chain Sprocket 26/RConn1 -- Simscape Bus/LConn26
  CF Chain Sprocket 27/RConn1 -- Simscape Bus/LConn27
  CF Chain Sprocket 28/RConn1 -- Simscape Bus/LConn28
  Simscape Bus/RConn1 -- F/RConn1
